simulink model "Izhikevich_QIF_Take2"  (R2019a)
settings: Solver=VariableStepAuto  StartTime=0.0  StopTime=500  RelTol=1e-9
values from neighbouring files (symbols this model uses):
  a = .02    (= 0.02)    [H_H_Mod.m]    (also in Part2.m)
  b = .2    (= 0.2)    [H_H_Mod.m]    (also in Part2.m)
  c = -50    [H_H_Mod.m]    (also in Part2.m = -65)
  d = 2    [H_H_Mod.m]    (also in Part2.m = 8)
  g = 1    [H_H_Mod.m]    (also in Part2.m = 10)
undefined symbols (not defined in the file or in its folder): sigbuilder_block
libraries: simulink x1
settings Model: Creator=Pranav Maddula  LastModifiedBy=Pranav Maddula

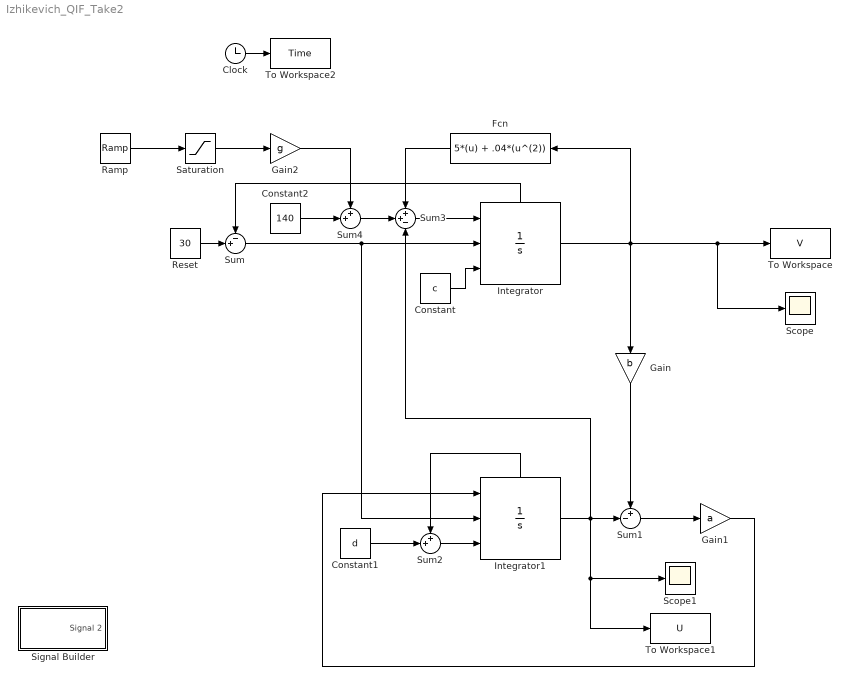
== system Izhikevich_QIF_Take2 ==
  Clock : Clock
  Constant : Constant  Value=c
  Constant1 : Constant  Value=d
  Constant2 : Constant  Value=140
  Fcn : Fcn  Expr=5*(u) + .04*(u^(2))
  Gain : Gain  Gain=b
  Gain1 : Gain  Gain=a
  Gain2 : Gain  Gain=g
  Integrator : Integrator  ExternalReset=falling  InitialConditionSource=external  ShowStatePort=on
  Integrator1 : Integrator  ExternalReset=falling  InitialConditionSource=external  ShowStatePort=on
  Ramp : simulink/Sources/Ramp  slope=0.1  start=1  InitialOutput=0
  Reset : Constant  Value=30
  Saturation : Saturate  UpperLimit=10  LowerLimit=0
  Scope : Scope
  Scope1 : Scope
  Signal Builder : Subsystem  Tag=STV Subsys  LoadFcn=sigbuilder_block('load');  StartFcn=sigbuilder_block('start');  StopFcn=sigbuilder_block('stop');  ClipboardFcn=sigbuilder_block('clipboard');  mask(Sigbuilder block){tuvar=[0:10]}
      mask help: Simulink:masks:SigbuilderBlock_MD
      mask init:
      | if ~strcmp(get_param(bdroot(gcbh),'SimulationStatus'),'stopped') tuvar = sigbuilder_block('maskInit'); end
      settings: CopyFcn=sigbuilder_block('copy');  DeleteFcn=sigbuilder_block('delete');  ModelCloseFcn=sigbuilder_block('modelClose');  PreSaveFcn=sigbuilder_block('preSave');  PauseFcn=sigbuilder_block('pause');  ContinueFcn=sigbuilder_block('continue');  NameChangeFcn=sigbuilder_block('namechange');  OpenFcn=sigbuilder_block('open',[437.6 199.2 550.4 400 ]);  CloseFcn=sigbuilder_block('close');
      mask Display: plot(0, 0, 100, 100,[2, 2, 32, 32, 2], [68, 8, 8, 68, 68],[32, 2], [38, 38], [32, 19, 2],[53, 60, 44], [32, 17, 17, 2],[16, 16, 31, 31]);txt = getActiveGroup(gcbh);text(2, 100, txt,'verticalAlignment', 'top');
  Sum : Sum  Inputs=-+|
  Sum1 : Sum  Inputs=+-|
  Sum2 : Sum  Inputs=++|
  Sum3 : Sum  Inputs=++-
  Sum4 : Sum  Inputs=++|
  To Workspace : ToWorkspace  VariableName=V  SampleTime=-1
  To Workspace1 : ToWorkspace  VariableName=U  SampleTime=-1
  To Workspace2 : ToWorkspace  VariableName=Time  SampleTime=-1
  wires:
  Reset/1 -> Sum/2
  Integrator/State -> Sum/1
  Constant/1 -> Integrator/3
  Sum/1 -> Integrator1/2, Integrator/2
  Integrator/1 -> Fcn/1, Gain/1, Scope/1, To Workspace/1
  Integrator1/1 -> Scope1/1, To Workspace1/1, Sum1/2, Sum3/3
  Gain/1 -> Sum1/1
  Sum1/1 -> Gain1/1
  Gain1/1 -> Integrator1/1
  Sum2/1 -> Integrator1/3
  Integrator1/State -> Sum2/1
  Constant1/1 -> Sum2/2
  Fcn/1 -> Sum3/1
  Sum3/1 -> Integrator/1
  Sum4/1 -> Sum3/2
  Constant2/1 -> Sum4/2
  Gain2/1 -> Sum4/1
  Clock/1 -> To Workspace2/1
  Saturation/1 -> Gain2/1
  Ramp/1 -> Saturation/1

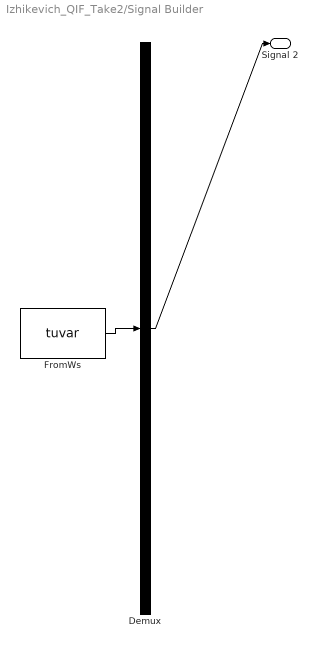
== system Izhikevich_QIF_Take2/Signal Builder ==
  Demux : Demux  Tag=STV Demux  Outputs=1
  FromWs : FromWorkspace  Tag=STV FromWs  VariableName=tuvar  SampleTime=0
      SigBuilderData=|
      | common.afterFinalStr = 'Extrapolate'
      | common.sampleTime = 0
      | dataSet.timeRange = [0 1100]
      | dataSet.name = 'Group 1'
      | sbobj.Groups.Name = 'Group 1'
      | sbobj.Groups.Signals.Name = 'Signal 2'
      | sbobj.Groups.Signals.XData = [0 1 1.01 600 1100]
      | sbobj.Groups.Signals.YData = [0 0 1 1 1]
      | sbobj.Groups.TimeRange = [0 1100]
  Signal 2 : Outport  Tag=STV Outport
  wires:
  FromWs/1 -> Demux/1
  Demux/1 -> Signal 2/1
